simulink model "EX_2_3_and_2_4_SL"  (R2018a)
settings: Solver=VariableStepAuto  StartTime=0.0  StopTime=10.0  RelTol=1e-3  EnableMultiTasking=on
settings Model: Creator=Andy  LastModifiedBy=Admin
settings DataIOCC: LimitDataPoints=on
settings OptimizationCC: LifeSpan=inf
settings DebuggingCC: AllowSymbolicDim=off  SFUnexpectedBacktrackingDiag=warning  SFNoUnconditionalDefaultTransitionDiag=warning  SFExecutionAtInitializationDiag=none
settings ModelReferenceCC: PropagateSignalLabelsOutOfModel=off
settings CodeAppCC: StateflowObjectComments=on
settings GRTTargetCC: TargetLangStandard=C89/C90 (ANSI)
settings ConfigComp: CovMetricSettings=dw  CovHtmlReporting=on  CovSaveCumulativeToWorkspaceVar=on  CovSaveSingleToWorkspaceVar=on  CovExternalEMLEnable=off

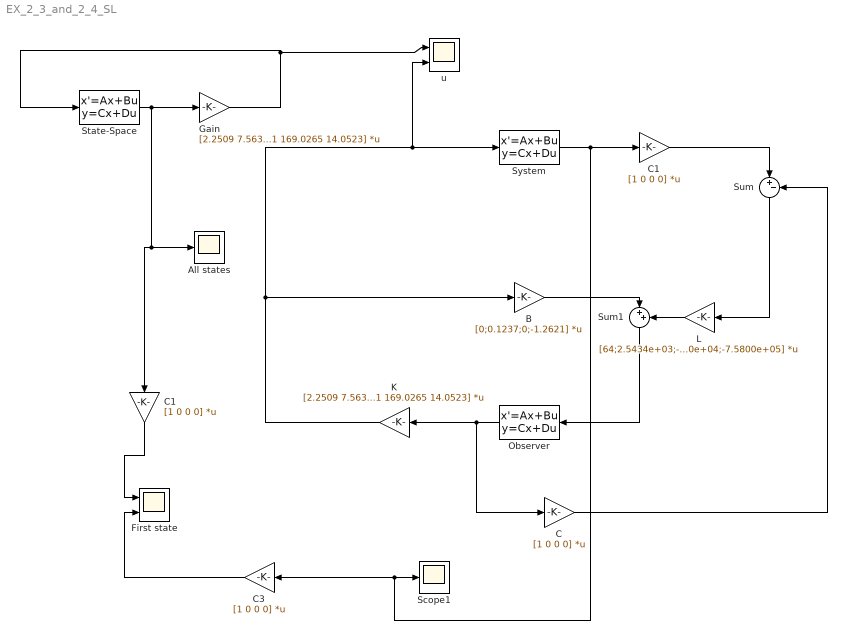
== system EX_2_3_and_2_4_SL ==
  All states : Scope
  B : Gain  Gain=[0;0.1237;0;-1.2621]  Multiplication=Matrix(K*u)
  C : Gain  Gain=[1 0 0 0]  Multiplication=Matrix(K*u)
  C1 : Gain  Gain=[1 0 0 0]  Multiplication=Matrix(K*u)
  "C1 " : Gain  Gain=[1 0 0 0]  Multiplication=Matrix(K*u)
  "C3 " : Gain  Gain=[1 0 0 0]  Multiplication=Matrix(K*u)
  First state : Scope  NumInputPorts=2
  Gain : Gain  Gain=[2.2509 7.5631 169.0265 14.0523]  Multiplication=Matrix(K*u)
  K : Gain  Gain=[2.2509 7.5631 169.0265 14.0523]  Multiplication=Matrix(K*u)
  L : Gain  Gain=[64;2.5434e+03;-5.1820e+04;-7.5800e+05]  Multiplication=Matrix(K*u)
  Observer : StateSpace  A=[0 1 0 0;0 0 -1 0;0 0 0 1;0 0 100 0]  B=eye(4)  C=eye(4)  D=zeros(4)  InitialCondition=[0;0;0.0;0]
  Scope1 : Scope
  State-Space : StateSpace  A=[0 1 0 0;0 0 -1 0;0 0 0 1;0 0 100 0]  B=[0;0.1237;0;-1.2621]  C=eye(4)  D=[0;0;0;0]  InitialCondition=[0;0;0.01;0]
  Sum : Sum  Inputs=|+-
  Sum1 : Sum  Inputs=|++
  "System " : StateSpace  A=[0 1 0 0;0 0 -1 0;0 0 0 1;0 0 100 0]  B=[0;0.1237;0;-1.2621]  C=eye(4)  D=[0;0;0;0]  InitialCondition=[0;0;0.01;0]
  u : Scope  NumInputPorts=2
  wires:
  State-Space/1 -> All states/1, C1/1, Gain/1
  Gain/1 -> u/1, State-Space/1
  "System "/1 -> "C3 "/1, Scope1/1, "C1 "/1
  Observer/1 -> C/1, K/1
  K/1 -> B/1, u/2, "System "/1
  B/1 -> Sum1/1
  L/1 -> Sum1/2
  Sum1/1 -> Observer/1
  Sum/1 -> L/1
  "C1 "/1 -> Sum/1
  C/1 -> Sum/2
  C1/1 -> First state/1
  "C3 "/1 -> First state/2
